simulink model "LinearModelAndLinearController"  (R2017a)
settings: Solver=ode4  StartTime=0.0  StopTime=time  FixedStep=time_steps  RelTol=1e-3
values from neighbouring files (symbols this model uses):
  A = [   0,0,1,0 ... (first row only)    [FeedbackGain.m]    (also in LinearisedModel.m = A_; integral_control.m; matlab.mat = 0.1621924326; nat_freq_stable_sys.m)
  B = [0;0;1/AA;1/FF]    [FeedbackGain.m]    (also in LinearisedModel.m; integral_control.m; matlab.mat = 0.0800927225; nat_freq_stable_sys.m)
  K = acker(A,B,pc)    [FeedbackGain.m]    (also in LinearisedModel.m = acker(A_,B,pc); integral_control.m; matlab.mat = 0; nat_freq_stable_sys.m = -f2)
  motor_stall_torque = 6    [LinearAnimations.m]    (also in LinearisedModel.m = 2.8; NonLinearAnimations.m = 1.36; experiment_vs_simulated.m = 8)
  q_start = [0;-pi/60;0;0]    [LinearisedModel.m]
settings Model: Creator=Henry  LastModifiedBy=Henry

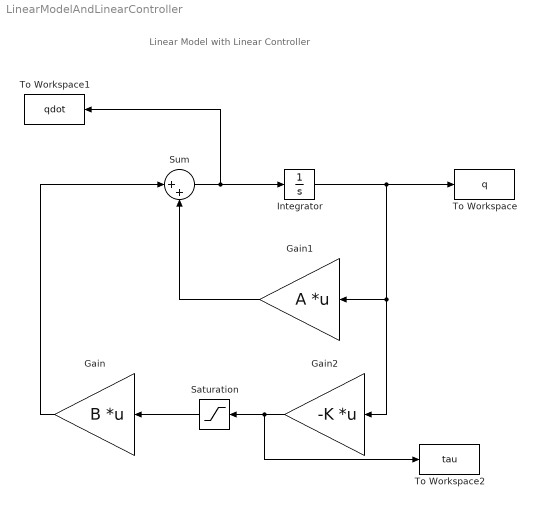
== system LinearModelAndLinearController ==
  note: Linear Model with Linear Controller
  Gain : Gain  Gain=B  Multiplication=Matrix(K*u)
  Gain1 : Gain  Gain=A  Multiplication=Matrix(K*u)  OutMin=[4]  OutMax=[4]
  Gain2 : Gain  Gain=-K  Multiplication=Matrix(K*u)
  Integrator : Integrator  InitialCondition=q_start
  Saturation : Saturate  UpperLimit=motor_stall_torque  LowerLimit=-1*motor_stall_torque
  Sum : Sum  Inputs=|++
  To Workspace : ToWorkspace  VariableName=q  SaveFormat=Timeseries  SampleTime=-1
  To Workspace1 : ToWorkspace  VariableName=qdot  SaveFormat=Timeseries  SampleTime=-1
  To Workspace2 : ToWorkspace  VariableName=tau  SaveFormat=Timeseries  SampleTime=-1
  wires:
  Sum/1 -> To Workspace1/1, Integrator/1
  Gain1/1 -> Sum/2
  Gain/1 -> Sum/1
  Integrator/1 -> Gain2/1, Gain1/1, To Workspace/1
  Gain2/1 -> To Workspace2/1, Saturation/1
  Saturation/1 -> Gain/1
